simulink model "HTSE_electrolyzer_1MW_DC"  (R2020b)
settings: Solver=ode15s  StartTime=0.0  StopTime=3600*1
model workspace: external: MAT-File (data not in the file)
values from neighbouring files (symbols this model uses):
  Acsflow_aHR = Ltubet * tubenodewidth_aHR    [Electrolyzer_load.m]
  Acsflow_wHR = Ltubet * tubenodewidth_wHR    [Electrolyzer_load.m]
  Anode_aHR = pi*Dtubeo*tubenodewidth_aHR*ntubes    (= 5.35151053616)    [Electrolyzer_load.m]
  Anode_wHR = pi*Dtubeo*tubenodewidth_wHR*ntubes    (= 2.79287586904)    [Electrolyzer_load.m]
  C1 = C1par(4,4)    [tubebankpar.m]
  Cp_I = 500    [Electrolyzer_load.m]
  Cp_S = 500    [Electrolyzer_load.m]
  Dtubei = 0.015748    [Electrolyzer_load.m]
  Dtubeo = Dtubei +2*ttube    (= 0.021336)    [Electrolyzer_load.m]
  dx_cell = L_cell/n_cell    (= 0.0125)    [Electrolyzer_load.m]
  eps_I = 0.1    [Electrolyzer_load.m]
  eps_S = 0.8    [Electrolyzer_load.m]
  F = 96485.33    [Electrolyzer_load.m]    (also in localcur.m = params(6*n+2))
  H2concSS = [9.66170610517 15.4200127744 21.0651099255 26.4111027106 31.267340431 36.180096143 39.6625030093 45.9597835644]    [concSS.mat]
  H2OconcSS = [46.3863122499 40.6280055806 34.9829084296 29.6369156445 24.7806779241 19.8679222121 16.3855153458 10.0882347907]    [concSS.mat]
  h_A = 0.001    [Electrolyzer_load.m]
  h_C = 0.001    [Electrolyzer_load.m]
  h_I = 7.5e-4    (= 0.00075)    [Electrolyzer_load.m]
  h_S = t_C + t_E + t_A    (= 0.00034)    [Electrolyzer_load.m]
  k_A = (Nu_A*lam_A)/dh_A    (= 107.851842105)    [Electrolyzer_load.m]
  k_C = (Nu_C*lam_C)/dh_C    (= 303.235614035)    [Electrolyzer_load.m]
  ktube = 60.5    [Electrolyzer_load.m]
  L_cell = 0.1    [Electrolyzer_load.m]
  lam_I = 25    [Electrolyzer_load.m]
  lam_S = 2    [Electrolyzer_load.m]
  m = mpar(4,4)    [tubebankpar.m]
  MM_H2 = 2    [Electrolyzer_load.m]
  MM_H2O = 18    [Electrolyzer_load.m]
  MM_N2 = 28    [Electrolyzer_load.m]
  MM_O2 = 32    [Electrolyzer_load.m]
  N2concSS = [42.0361226095 42.0361226095 42.0361226095 42.0361226095 42.0361226095 42.0361226095 42.0361226095 42.0361226095]    [concSS.mat]
  n_cell = 8    [Electrolyzer_load.m]
  nhx_aHR = 31    [Electrolyzer_load.m]
  nhx_wHR = 15    [Electrolyzer_load.m]
  ntubes = 500    [Electrolyzer_load.m]
  num_cells = 605711/100    (= 6057.11)    [Electrolyzer_load.m]
  O2concSS = [15.418006168 17.4148227344 19.3723814677 21.2262193353 22.9102241109 24.6138277145 25.8214271218 28.005144464]    [concSS.mat]
  Ppa = 5e5    (= 500000)    [Electrolyzer_load.m]
  rho_I = 8000    [Electrolyzer_load.m]
  rho_S = 5900    [Electrolyzer_load.m]
  sig = 5.6703e-8    (= 5.6703e-08)    [Electrolyzer_load.m]
  St = StD*Dtubeo    (= 0.042672)    [Electrolyzer_load.m]
  T_aSHout = 700 + 273.13    (= 973.13)    [Electrolyzer_load.m]
  T_cell_init = 1073    [Electrolyzer_load.m]
  T_wSHout = 700 + 273.13    (= 973.13)    [Electrolyzer_load.m]
  ttube = 0.002794    [Electrolyzer_load.m]
  V_shell_aHR = (Acsflow_aHR*Ltubel) - (pi*(Dtubeo/2)^2*tubenodewidth_aHR*ntubes)    [Electrolyzer_load.m]
  V_shell_wHR = (Acsflow_wHR*Ltubel) - (pi*(Dtubeo/2)^2*tubenodewidth_wHR*ntubes)    [Electrolyzer_load.m]
  V_tubes_aHR = pi*(Dtubei/2)^2*tubenodewidth_aHR*ntubes    (= 0.0155508525335)    [Electrolyzer_load.m]
  V_tubes_wHR = pi*(Dtubei/2)^2*tubenodewidth_wHR*ntubes    (= 0.00811576479021)    [Electrolyzer_load.m]
  W_cell = 0.0855    [Electrolyzer_load.m]
  x0 = zeros((5*n_cell),1)    [Electrolyzer_load.m]    (also in eqsolver.m = zeros((5*n),1))
libraries: pid_lib x1
settings Model: Creator=jimmonen  LastModifiedBy=jimmonen

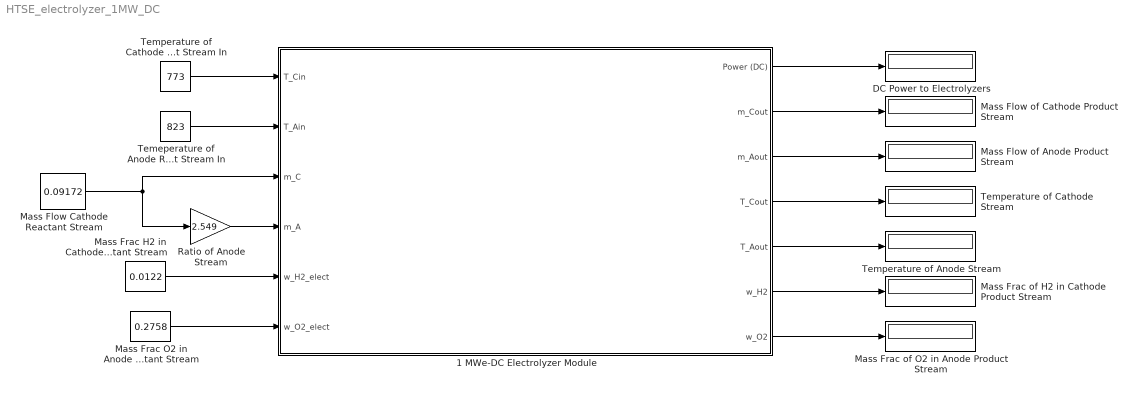
== system HTSE_electrolyzer_1MW_DC ==
  1 MWe-DC Electrolyzer Module : Subsystem
      mask Display: image('G:\My Drive\3. Research\6. HTSE - Detailed Plant\Paper\Figures\SH-FHTSE-1 MW Module.drawio.png'); % Use "Edit Image" on toolstrip to change.
  DC Power to Electrolyzers : Display
  Mass Flow Cathode Reactant Stream : Constant  Value=0.09172
  Mass Flow of Anode Product Stream : Display
  Mass Flow of Cathode Product Stream : Display
  Mass Frac H2 in Cathode Reactant Stream : Constant  Value=0.0122
  Mass Frac O2 in Anode Reactant Stream : Constant  Value=0.2758
  Mass Frac of H2 in Cathode Product Stream : Display
  Mass Frac of O2 in Anode Product Stream : Display
  Ratio of Anode Stream : Gain  Gain=2.549
  Temeperature of Anode Reactant Stream In : Constant  Value=823
  Temperature of Anode Stream : Display
  Temperature of Cathode Reactant Stream In : Constant  Value=773
  Temperature of Cathode Stream : Display
  wires:
  Mass Frac H2 in Cathode Reactant Stream/1 -> 1 MWe-DC Electrolyzer Module/5(w_H2_elect)
  Mass Frac O2 in Anode Reactant Stream/1 -> 1 MWe-DC Electrolyzer Module/6(w_O2_elect)
  Ratio of Anode Stream/1 -> 1 MWe-DC Electrolyzer Module/4(m_A)
  Temperature of Cathode Reactant Stream In/1 -> 1 MWe-DC Electrolyzer Module/1(T_Cin)
  Mass Flow Cathode Reactant Stream/1 -> Ratio of Anode Stream/1, 1 MWe-DC Electrolyzer Module/3(m_C)
  Temeperature of Anode Reactant Stream In/1 -> 1 MWe-DC Electrolyzer Module/2(T_Ain)
  1 MWe-DC Electrolyzer Module/1(Power (DC)) -> DC Power to Electrolyzers/1
  1 MWe-DC Electrolyzer Module/2(m_Cout) -> Mass Flow of Cathode Product Stream/1
  1 MWe-DC Electrolyzer Module/3(m_Aout) -> Mass Flow of Anode Product Stream/1
  1 MWe-DC Electrolyzer Module/6(w_H2) -> Mass Frac of H2 in Cathode Product Stream/1
  1 MWe-DC Electrolyzer Module/7(w_O2) -> Mass Frac of O2 in Anode Product Stream/1
  1 MWe-DC Electrolyzer Module/4(T_Cout) -> Temperature of Cathode Stream/1
  1 MWe-DC Electrolyzer Module/5(T_Aout) -> Temperature of Anode Stream/1

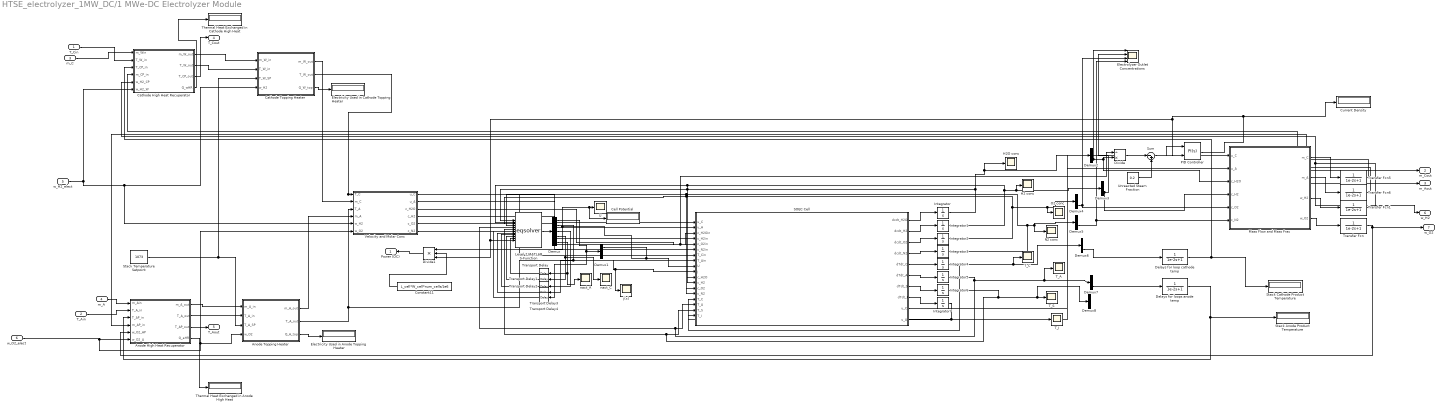
== system HTSE_electrolyzer_1MW_DC/1 MWe-DC Electrolyzer Module ==
  T_Cin : Inport
  T_Ain : Inport  Port=2
  m_C : Inport  Port=3
  m_A : Inport  Port=4
  w_H2_elect : Inport  Port=5
  w_O2_elect : Inport  Port=6
  " SOEC Cell" : MATLAB Function  TreatAsAtomicUnit=on
  Anode High Heat Recuperator : Subsystem
  Anode Topping Heater : MATLAB Function  TreatAsAtomicUnit=on
  Cathode High Heat Recuperator : Subsystem
  Cathode Topping Heater : MATLAB Function  TreatAsAtomicUnit=on
  Cell Potential : Display
  Constant11 : Constant  Value=L_cell*W_cell*num_cells/1e6
  Current Density : Display
  Delays for loop cathode temp : TransferFcn  Denominator=[1e-2 1]
  Delays for loops anode temp : TransferFcn  Denominator=[1e-2 1]
  Demux : Demux  Outputs=[n_cell n_cell n_cell n_cell n_cell ]
  Demux1 : Demux  Outputs=[1 n_cell-1]
  Demux{2..8} (7 alike) : Demux  Outputs=[n_cell-1 1]
  Divide : Product  Inputs=/*
  Divide1 : Product  Inputs=***
  Electricity Used in Anode Topping Heater : Display
  Electricity Used in Cathode Topping Heater : Display
  Electrolyzer Outlet Concentrations : Scope  NumInputPorts=4
  H2 conc : Scope
  H2O conc : Scope
  Integrator : Integrator  InitialCondition=H2OconcSS
  Integrator1 : Integrator  InitialCondition=H2concSS
  Integrator2 : Integrator  InitialCondition=O2concSS
  Integrator3 : Integrator  InitialCondition=N2concSS
  Integrator{4..7} (4 alike) : Integrator  InitialCondition=T_cell_init*ones(n_cell,1)
  Level-2 MATLAB S-Function : M-S-Function  FunctionName=eqsolver  Parameters=n_cell, F, R, t_C, t_E, t_A, sig_C, sig_A, sig_E, A_C, A_A, E_C, E_A, Deff_C, Deff_A, alph, Ppa
  Mass Flow and Mass Frac : MATLAB Function  TreatAsAtomicUnit=on
  N2 conc : Scope
  O2 conc : Scope
  PID Controller : pid_lib/PID Controller  Controller=PI  Form=Parallel  TimeDomain=Continuous-time  UseExternalTs=off  SampleTime=-1  IntegratorMethod=Forward Euler  FilterMethod=Forward Euler  ControllerParametersSource=internal  P=30  I=-12.5  D=0  UseFilter=on  N=100  TunerSelectOption=Transfer Function Based (PID Tuner App)  InitialConditionSource=internal  InitialConditionForIntegrator=15000  InitialConditionForFilter=0  DifferentiatorICPrevScaledInput=0  ExternalReset=none  TrackingMode=on  Kt=1  LimitOutput=on  SatLimitsSource=internal  UpperSaturationLimit=15000  LowerSaturationLimit=0  LinearizeAsGain=on  AntiWindupMode=none  Kb=1  POutMin=[]  POutMax=[]  IOutMin=[]  IOutMax=[]  DOutMin=[]  DOutMax=[]  NOutMin=[]  NOutMax=[]  SumOutMin=[]  SumOutMax=[]  SaturationOutMin=[]  SaturationOutMax=[]  PParamMin=[]  PParamMax=[]  IParamMin=[]  IParamMax=[]  DParamMin=[]  DParamMax=[]  NParamMin=[]  NParamMax=[]  KbParamMin=[]  KbParamMax=[]  KtParamMin=[]  KtParamMax=[]  KbOutMin=[]  KbOutMax=[]  KtOutMin=[]  KtOutMax=[]  IntegratorOutMin=[]  IntegratorOutMax=[]  FilterOutMin=[]  FilterOutMax=[]  SumI1OutMin=[]  SumI1OutMax=[]  SumI2OutMin=[]  SumI2OutMax=[]  SumI3OutMin=[]  SumI3OutMax=[]  SumI4OutMin=[]  SumI4OutMax=[]  SumDOutMin=[]  SumDOutMax=[]  DifferentiatorOutMin=[]  DifferentiatorOutMax=[]  FilterDiffOutCoefMin=[]  FilterDiffOutCoefMax=[]  ReciprocalOutMin=[]  ReciprocalOutMax=[]  SumDenOutMin=[]  SumDenOutMax=[]  SumNumOutMin=[]  SumNumOutMax=[]  DivideOutMin=[]  DivideOutMax=[]  UdiffTsProdOutMin=[]  UdiffTsProdOutMax=[]  NTsProdOutMin=[]  NTsProdOutMax=[]  UintegralTsProdOutMin=[]  UintegralTsProdOutMax=[]  UngainTsProdOutMin=[]  UngainTsProdOutMax=[]  IntegratorContinuousStateAttributes=''  IntegratorStateMustResolveToSignalObject=off  IntegratorRTWStateStorageClass=Auto  FilterContinuousStateAttributes=''  FilterStateMustResolveToSignalObject=off  FilterRTWStateStorageClass=Auto  ParallelPVariant=InternalParameters  IdealPVariant=Disabled  IVariant=InternalParameters  DVariant=Disabled  IntegratorVariant=Continuous  SatVariant=Enabled  AWVariant=Passthrough  PCopyVariant=Disabled  TRVariant=Enabled  FdbkBlocksVariant=Forward  IdealPFdbkVariant=Disabled  SatFdbkVariant=Disabled  DerivativeFilterVariant=Disabled  NVariant=Disabled  NCopyVariant=Disabled_SignalSpec  FilterICVariant=Disabled  IntegratorICVariant=InternalICs  ExternalResetVariant=Disabled  TRSumVariant=TrackingMode  SumFdbkVariant=Disabled  SumVariant=Sum_PI  TsampFilterVariant=InternalTs  TsampNgainVariant=Passthrough  TsampIntegralVariant=Passthrough  ExternalSaturationOutDataTypeStr=Inherit: Same as second input
  Stack Anode Product Temperature : Display
  Stack Cathode Product Temperature : Display
  Stack Temperature Setpoint : Constant  Value=1073
  Sum : Sum  Inputs=|-+
  T_A : Scope
  T_C : Scope
  T_I : Scope
  T_S : Scope
  Thermal Heat Exchanged in Anode High Heat : Display
  Thermal Heat Exchanged in Cathode High Heat : Display
  Transfer Fcn{,1,5..6} (4 alike) : TransferFcn  Denominator=[1e-2 1]
  Transport Delay : TransportDelay  DelayTime=0.1  InitialOutput=x0(4*n_cell+1:end)
  Transport Delay1 : TransportDelay  DelayTime=0.1  InitialOutput=x0(3*n_cell+1:4*n_cell)
  Transport Delay2 : TransportDelay  DelayTime=0.1  InitialOutput=x0(2*n_cell+1:3*n_cell)
  Transport Delay3 : TransportDelay  DelayTime=0.1  InitialOutput=x0(n_cell+1:2*n_cell)
  Transport Delay4 : TransportDelay  DelayTime=0.1  InitialOutput=x0(1:n_cell)
  U : Scope
  Unreacted Steam Fraction : Constant  Value=0.2
  Velocity and Molar Conc : MATLAB Function  TreatAsAtomicUnit=on
  j(x) : Scope
  nact_A : Scope
  nact_C : Scope
  Power (DC) : Outport
  m_Cout : Outport  Port=2
  m_Aout : Outport  Port=3
  T_Cout : Outport  Port=4
  T_Aout : Outport  Port=5
  w_H2 : Outport  Port=6
  w_O2 : Outport  Port=7
  wires:
  " SOEC Cell"/2(dcdt_H2) -> Integrator1/1
  " SOEC Cell"/7(dTdt_S) -> Integrator6/1
  " SOEC Cell"/3(dcdt_O2) -> Integrator2/1
  Divide1/1 -> Power (DC)/1
  " SOEC Cell"/5(dTdt_C) -> Integrator4/1
  Demux6/2 -> Delays for loop cathode temp/1
  Integrator4/1 -> Demux6/1, T_C/1, " SOEC Cell"/15(T_C)
  Integrator7/1 -> " SOEC Cell"/18(T_I), T_I/1
  " SOEC Cell"/8(dTdt_I) -> Integrator7/1
  Demux2/2 -> Divide/2, Mass Flow and Mass Frac/3(c_H2O), Electrolyzer Outlet Concentrations/1
  " SOEC Cell"/4(dcdt_N2) -> Integrator3/1
  " SOEC Cell"/6(dTdt_A) -> Integrator5/1
  Divide/1 -> Sum/1
  Sum/1 -> PID Controller/1
  Constant11/1 -> Divide1/2
  Demux7/2 -> Delays for loops anode temp/1
  " SOEC Cell"/1(dcdt_H2O) -> Integrator/1
  Demux4/2 -> Electrolyzer Outlet Concentrations/3, Mass Flow and Mass Frac/5(c_O2)
  Demux5/2 -> Electrolyzer Outlet Concentrations/4, Mass Flow and Mass Frac/6(c_N2)
  Mass Flow and Mass Frac/1(m_C) -> Transfer Fcn5/1
  Mass Flow and Mass Frac/2(m_A) -> Transfer Fcn6/1
  " SOEC Cell"/9(u_C) -> Mass Flow and Mass Frac/1(u_C)
  " SOEC Cell"/10(u_A) -> Mass Flow and Mass Frac/2(u_A)
  Mass Flow and Mass Frac/4(w_O2) -> Transfer Fcn/1
  Mass Flow and Mass Frac/3(w_H2) -> Transfer Fcn1/1
  w_H2_elect/1 -> Cathode Topping Heater/4(w_H2), Velocity and Molar Conc/5(w_H2), Cathode High Heat Recuperator/6(w_H2_W)
  w_O2_elect/1 -> Velocity and Molar Conc/6(w_O2), Anode Topping Heater/4(w_O2), Anode High Heat Recuperator/6(w_O2_A)
  Velocity and Molar Conc/1(u_C) -> " SOEC Cell"/1("u_C ")
  Velocity and Molar Conc/2(u_A) -> " SOEC Cell"/2("u_A ")
  Velocity and Molar Conc/3(c_H2O) -> Divide/1, " SOEC Cell"/3(c_H2Oin)
  Velocity and Molar Conc/4(c_H2) -> " SOEC Cell"/4(c_H2in)
  Velocity and Molar Conc/5(c_O2) -> " SOEC Cell"/5(c_O2in)
  Velocity and Molar Conc/6(c_N2) -> " SOEC Cell"/6(c_N2in)
  Transfer Fcn/1 -> Anode High Heat Recuperator/5(w_O2_AP), w_O2/1
  Transfer Fcn1/1 -> w_H2/1, Cathode High Heat Recuperator/5(w_H2_CP)
  Demux/2 -> Transport Delay3/1, " SOEC Cell"/10(j), j(x)/1
  Integrator1/1 -> Level-2 MATLAB S-Function/2, " SOEC Cell"/12(c_H2), Demux3/1, H2 conc/1
  Integrator/1 -> Demux2/1, H2O conc/1, Level-2 MATLAB S-Function/1, " SOEC Cell"/11(c_H2O)
  Transport Delay3/1 -> Level-2 MATLAB S-Function/8
  Demux/3 -> Transport Delay2/1
  Demux/1 -> Transport Delay4/1, Demux1/1
  Integrator5/1 -> Level-2 MATLAB S-Function/5, " SOEC Cell"/16(T_A), Demux7/1, T_A/1
  Level-2 MATLAB S-Function/1 -> Demux/1
  Demux/5 -> Transport Delay/1, nact_A/1
  Demux/4 -> Transport Delay1/1, nact_C/1
  Transport Delay2/1 -> Level-2 MATLAB S-Function/9
  Transport Delay4/1 -> Level-2 MATLAB S-Function/7
  Transport Delay1/1 -> Level-2 MATLAB S-Function/10
  Transport Delay/1 -> Level-2 MATLAB S-Function/11
  Integrator2/1 -> Level-2 MATLAB S-Function/3, " SOEC Cell"/13(c_O2), Demux4/1, O2 conc/1
  Demux1/1 -> Cell Potential/1, U/1, Divide1/1, " SOEC Cell"/9(U)
  Demux3/2 -> Electrolyzer Outlet Concentrations/2, Mass Flow and Mass Frac/4(c_H2)
  Cathode High Heat Recuperator/2(T_W_out) -> Cathode Topping Heater/2(T_W_in)
  Cathode High Heat Recuperator/1(m_W_out) -> Cathode Topping Heater/1(m_W_in)
  Stack Temperature Setpoint/1 -> Anode Topping Heater/3(T_A_SP), Cathode Topping Heater/3(T_W_SP)
  m_C/1 -> Cathode High Heat Recuperator/1("m_Win ")
  T_Cin/1 -> Cathode High Heat Recuperator/2(T_W_in)
  Cathode Topping Heater/1(m_W_out) -> Velocity and Molar Conc/2(m_C)
  m_A/1 -> Anode High Heat Recuperator/1("m_Ain ")
  T_Ain/1 -> Anode High Heat Recuperator/2(T_A_in)
  Anode Topping Heater/1(m_A_out) -> Velocity and Molar Conc/4(m_A)
  Anode Topping Heater/2(T_A_out) -> Velocity and Molar Conc/3(T_A), " SOEC Cell"/8(T_Ain)
  Anode High Heat Recuperator/1(m_A_out) -> Anode Topping Heater/1(m_A_in)
  Delays for loop cathode temp/1 -> Cathode High Heat Recuperator/3(T_CP_in), Stack Cathode Product Temperature/1
  Delays for loops anode temp/1 -> Stack Anode Product Temperature/1, Anode High Heat Recuperator/3(T_AP_in)
  Transfer Fcn5/1 -> m_Cout/1, Cathode High Heat Recuperator/4("m_CP_in ")
  Transfer Fcn6/1 -> m_Aout/1, Anode High Heat Recuperator/4("m_AP_in ")
  PID Controller/1 -> PID Controller/2, Level-2 MATLAB S-Function/12, Divide1/3, Current Density/1
  Unreacted Steam Fraction/1 -> Sum/2
  Integrator6/1 -> Demux8/1, T_S/1, Level-2 MATLAB S-Function/6, " SOEC Cell"/17(T_S)
  Cathode Topping Heater/2(T_W_out) -> " SOEC Cell"/7(T_Cin), Velocity and Molar Conc/1(T_C)
  Integrator3/1 -> Demux5/1, N2 conc/1, Level-2 MATLAB S-Function/4, " SOEC Cell"/14(c_N2)
  Anode High Heat Recuperator/2(T_A_out) -> Anode Topping Heater/2(T_A_in)
  Cathode High Heat Recuperator/3(T_CP_out) -> T_Cout/1
  Cathode High Heat Recuperator/4(Q_wHR) -> Thermal Heat Exchanged in Cathode High Heat/1
  Cathode Topping Heater/3(Q_W_top) -> Electricity Used in Cathode Topping Heater/1
  Anode Topping Heater/3(Q_A_top) -> Electricity Used in Anode Topping Heater/1
  Anode High Heat Recuperator/3(T_AP_out) -> T_Aout/1
  Anode High Heat Recuperator/4(Q_aHR) -> Thermal Heat Exchanged in Anode High Heat/1

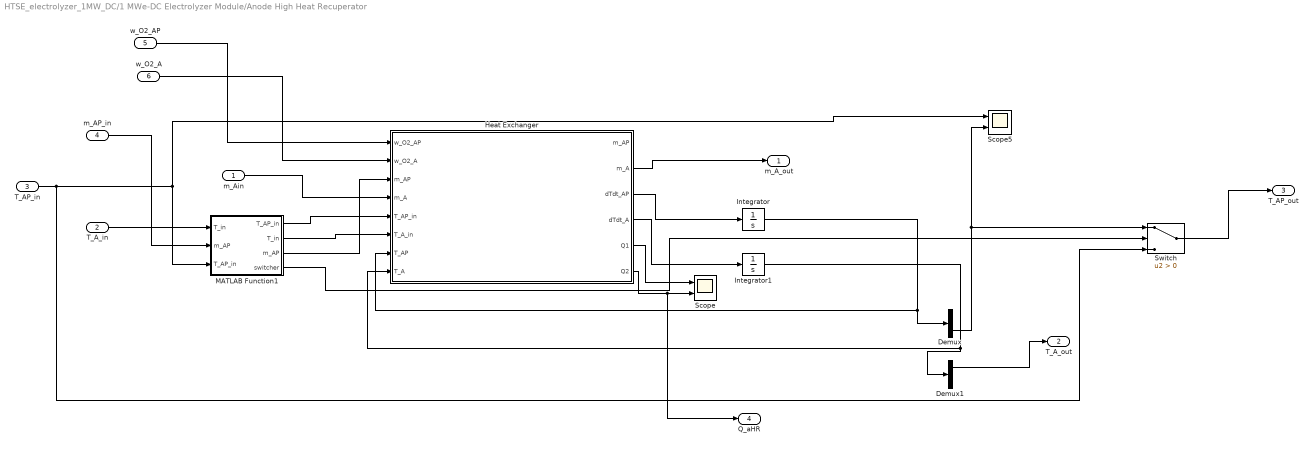
== system HTSE_electrolyzer_1MW_DC/1 MWe-DC Electrolyzer Module/Anode High Heat Recuperator ==
  "m_Ain " : Inport
  T_A_in : Inport  Port=2
  T_AP_in : Inport  Port=3
  "m_AP_in " : Inport  Port=4
  w_O2_AP : Inport  Port=5
  w_O2_A : Inport  Port=6
  Demux : Demux  Outputs=[nhx_aHR-1 1]
  Demux1 : Demux  Outputs=[1 nhx_aHR-1]
  Heat Exchanger : MATLAB Function  TreatAsAtomicUnit=on
  Integrator : Integrator  InitialCondition=ones(nhx_aHR, 1)*(T_aSHout)
  Integrator1 : Integrator  InitialCondition=ones(nhx_aHR, 1)*(T_aSHout)
  MATLAB Function1 : MATLAB Function  TreatAsAtomicUnit=on
  Scope : Scope  NumInputPorts=2
  Scope5 : Scope  NumInputPorts=2
  Switch : Switch  Criteria=u2 > Threshold
  m_A_out : Outport
  T_A_out : Outport  Port=2
  T_AP_out : Outport  Port=3
  Q_aHR : Outport  Port=4
  wires:
  Integrator1/1 -> Demux1/1, Heat Exchanger/8(T_A)
  "m_AP_in "/1 -> MATLAB Function1/2("m_AP ")
  Demux/2 -> Scope5/2, Switch/1
  Integrator/1 -> Demux/1, Heat Exchanger/7(T_AP)
  "m_Ain "/1 -> Heat Exchanger/4("m_A ")
  Heat Exchanger/4(dTdt_A) -> Integrator1/1
  Heat Exchanger/3(dTdt_AP) -> Integrator/1
  T_AP_in/1 -> Switch/3, Scope5/1, MATLAB Function1/3("T_AP_in ")
  Heat Exchanger/5(Q1) -> Scope/1
  MATLAB Function1/3(m_AP) -> Heat Exchanger/3("m_AP ")
  MATLAB Function1/2(T_in) -> Heat Exchanger/6(T_A_in)
  MATLAB Function1/1(T_AP_in) -> Heat Exchanger/5(T_AP_in)
  Demux1/1 -> T_A_out/1
  T_A_in/1 -> MATLAB Function1/1("T_in ")
  MATLAB Function1/4(switcher) -> Switch/2
  Switch/1 -> T_AP_out/1
  Heat Exchanger/6(Q2) -> Q_aHR/1, Scope/2
  Heat Exchanger/2(m_A) -> m_A_out/1
  w_O2_AP/1 -> Heat Exchanger/1(w_O2_AP)
  w_O2_A/1 -> Heat Exchanger/2(w_O2_A)

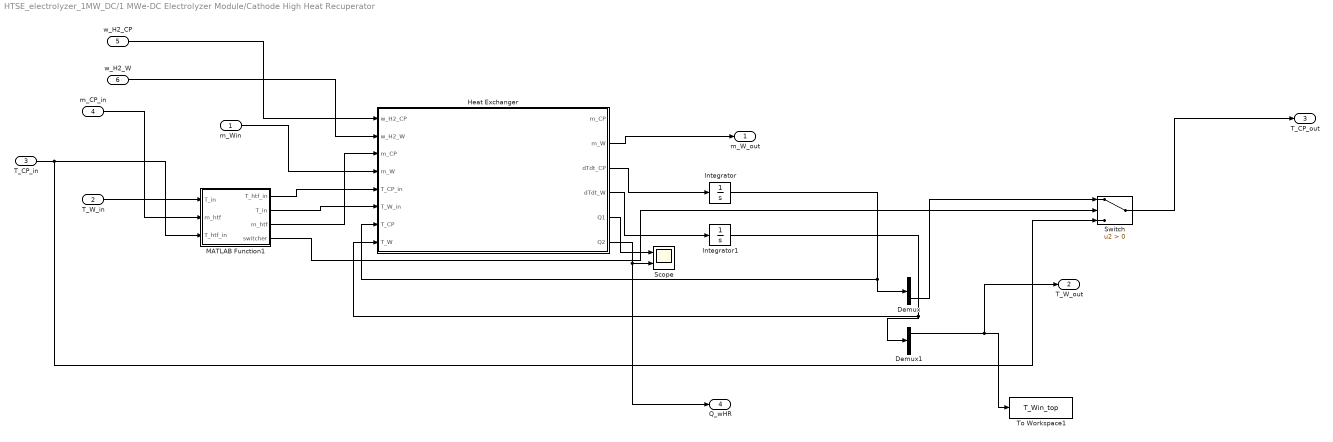
== system HTSE_electrolyzer_1MW_DC/1 MWe-DC Electrolyzer Module/Cathode High Heat Recuperator ==
  "m_Win " : Inport
  T_W_in : Inport  Port=2
  T_CP_in : Inport  Port=3
  "m_CP_in " : Inport  Port=4
  w_H2_CP : Inport  Port=5
  w_H2_W : Inport  Port=6
  Demux : Demux  Outputs=[nhx_wHR-1 1]
  Demux1 : Demux  Outputs=[1 nhx_wHR-1]
  Heat Exchanger : MATLAB Function  TreatAsAtomicUnit=on
  Integrator : Integrator  InitialCondition=ones(nhx_wHR, 1)*(T_wSHout)
  Integrator1 : Integrator  InitialCondition=ones(nhx_wHR, 1)*(T_wSHout)
  MATLAB Function1 : MATLAB Function  TreatAsAtomicUnit=on
  Scope : Scope  NumInputPorts=2
  Switch : Switch  Criteria=u2 > Threshold
  To Workspace1 : ToWorkspace  VariableName=T_Win_top  SaveFormat=Timeseries  SampleTime=-1
  m_W_out : Outport
  T_W_out : Outport  Port=2
  T_CP_out : Outport  Port=3
  Q_wHR : Outport  Port=4
  wires:
  Integrator1/1 -> Demux1/1, Heat Exchanger/8(T_W)
  "m_CP_in "/1 -> MATLAB Function1/2("m_htf ")
  Demux/2 -> Switch/1
  Integrator/1 -> Demux/1, Heat Exchanger/7(T_CP)
  "m_Win "/1 -> Heat Exchanger/4("m_W ")
  Heat Exchanger/4(dTdt_W) -> Integrator1/1
  Heat Exchanger/3(dTdt_CP) -> Integrator/1
  T_CP_in/1 -> Switch/3, MATLAB Function1/3("T_htf_in ")
  Heat Exchanger/5(Q1) -> Scope/1
  MATLAB Function1/3(m_htf) -> Heat Exchanger/3("m_CP ")
  MATLAB Function1/2(T_in) -> Heat Exchanger/6(T_W_in)
  MATLAB Function1/1(T_htf_in) -> Heat Exchanger/5(T_CP_in)
  Demux1/1 -> T_W_out/1, To Workspace1/1
  T_W_in/1 -> MATLAB Function1/1("T_in ")
  MATLAB Function1/4(switcher) -> Switch/2
  Switch/1 -> T_CP_out/1
  Heat Exchanger/6(Q2) -> Q_wHR/1, Scope/2
  Heat Exchanger/2(m_W) -> m_W_out/1
  w_H2_CP/1 -> Heat Exchanger/1(w_H2_CP)
  w_H2_W/1 -> Heat Exchanger/2(w_H2_W)

== matlab function HTSE_electrolyzer_1MW_DC/1 MWe-DC Electrolyzer Module/Mass Flow and Mass Frac ==
  data: u_C input; u_A input; c_H2O input; c_H2 input; c_O2 input; c_N2 input; num_cells parameter; MM_H2O parameter; h_A parameter; W_cell parameter; h_C parameter; MM_O2 parameter; m_C output; m_A output; w_H2 output; MM_N2 parameter; MM_H2 parameter; w_O2 output
function [m_C, m_A, w_H2, w_O2] = conc_to_mass(u_C, u_A, c_H2O, c_H2, c_O2, c_N2, num_cells, MM_H2O,h_A, W_cell, h_C, MM_O2, MM_N2, MM_H2)

%mass flows cathode
m_H2O = u_C*h_C*W_cell*MM_H2O*c_H2O*num_cells/1000;
m_H2 =  u_C*h_C*W_cell*MM_H2*c_H2*num_cells/1000;
m_C = m_H2O + m_H2;


%mass fractions cathode
w_H2O = m_H2O/(m_H2O + m_H2);
w_H2 = 1 - w_H2O;

%mass flows anode
m_O2 = u_A*h_A*W_cell*MM_O2*c_O2*num_cells/1000;
m_N2 = u_A*h_A*W_cell*MM_N2*c_N2*num_cells/1000;
m_A = (m_O2 + m_N2);

%mass fractions anode
w_O2 = m_O2/(m_O2 + m_N2);

== matlab function HTSE_electrolyzer_1MW_DC/1 MWe-DC Electrolyzer Module/Cathode High Heat Recuperator/Heat Exchanger ==
  data: w_H2_CP input; w_H2_W input; m_CP input; m_W input; T_CP_in input; T_W_in input; T_CP input; m_CP output; m_W output; T_W input; dTdt_CP output; dTdt_W output; V_shell_wHR parameter; V_tubes_wHR parameter; nhx_wHR parameter; Acsflow_wHR parameter; St parameter; Dtubei parameter; ntubes parameter; C1 parameter; m parameter; ktube parameter; ttube parameter; Dtubeo parameter; Anode_wHR parameter; Q1 output; Q2 output
function [m_CP, m_W, dTdt_CP, dTdt_W, Q1, Q2]   = HX(w_H2_CP, w_H2_W, m_CP, m_W, T_CP_in,  ...
    T_W_in, T_CP, T_W, V_shell_wHR, V_tubes_wHR, nhx_wHR,...
    Acsflow_wHR, St, Dtubei, ntubes, C1, m, ktube, ttube, Dtubeo, Anode_wHR)

%% Properties

T_CP_avg = (T_CP_in + T_CP(end))/2;
w_H2O_CP = 1 - w_H2_CP;

[rho_H2O1, mu_H2O1, k_H2O1, C_H2O1] = water(T_CP_avg);
[rho_H21, mu_H21, k_H21, C_H21] = hydrogen(T_CP_avg);

%use weight fractions for mixing of properties
[rho_CP, mu_CP, k_CP, C_CP] = prop_mix(rho_H2O1, rho_H21, mu_H2O1, mu_H21, k_H2O1, k_H21, C_H2O1, C_H21, w_H2O_CP, w_H2_CP);

% Steam Properties
T_W_avg = (T_W_in + T_W(1))/2;
w_H2O_W = 1 - w_H2_W;

[rho_H2O2, mu_H2O2, k_H2O2, C_H2O2] = water(T_W_avg);
[rho_H22, mu_H22, k_H22, C_H22] = hydrogen(T_W_avg);

%use weight fractions for mixing of properties
[rho_W, mu_W, k_W, C_W] = prop_mix(rho_H2O2, rho_H22, mu_H2O2, mu_H22, k_H2O2, k_H22, C_H2O2, C_H22, w_H2O_W, w_H2_W);


%% Heat Transfer Coefficient Calcs

%CP is in shell

Pr_CP = C_CP*mu_CP/k_CP; %Prandtl # for CP, flow in pipe

%Determining the Reynolds # of the HTF using the maximum velocity through
%bank of tubes
v_CP = m_CP/(Acsflow_wHR*rho_CP); %m/s, velocity before hitting any tubes
vmax_CP = (St*v_CP)/(St-Dtubeo);
Remax_CP = (rho_CP*vmax_CP*Dtubeo)/mu_CP; %max reynolds number based on diameter and flow in between tubes
Nu_CP = 1.13*C1 * Remax_CP^m * Pr_CP^(1/3);

h_CP = Nu_CP*k_CP/Dtubeo; %convection ht coefficient for htf in crossflow over a bank of tubes
                            %W/m^2*K

%==========================================================================
% Steam is in tubes

m_W = m_W/ntubes; %kg/s, divide flow up into each tube for Re calcs

v_W = m_W/(rho_W*pi*(Dtubei/2)^2);
Re_W = (rho_W*v_W*Dtubei)/mu_W; %Reynolds # for HTF, flow in pipe
Pr_W = C_W*mu_W/k_W; %Prandtl # for HTF, flow in pipe

%HT coef for turbulent flow in ciruclar tube, i.e. high Re#
h_W = 0.023*Re_W^0.8*Pr_W^0.4*k_W/(Dtubei); %W/(m^2*K)

%HT coef for laminar flow
if Re_W < 2000
    h_W = 4.36*k_W/(Dtubei); %W/(m^2*K)
end

%to be used in energy bal/ODE on HTF
%from Incroprera et al., pg 507&514


%calculating overall heat transfer coefficient using thermal resistance,
%ignores effects of fins and fouling

U = ( (1/h_CP) + (1/h_W) + (ttube/ktube) )^-1; %overall ht coef, W/m^2*K 

%% Energy Balance

%initializing each energybal as zero to define size of each column vector

dTdt_CP = zeros(size(T_CP));
dTdt_W = zeros(size(T_W));

%HTF energy balance
dTdt_CP(1) = (m_CP*C_CP*(T_CP_in - T_CP(1)) - U*Anode_wHR * (T_CP(1) - T_W(1)))/(V_shell_wHR*rho_CP*C_CP);
dTdt_CP(2:nhx_wHR) = (m_CP*C_CP*(T_CP(1:nhx_wHR-1) - T_CP(2:nhx_wHR)) - U*Anode_wHR * (T_CP(2:nhx_wHR) - T_W(2:nhx_wHR)))/(V_shell_wHR*rho_CP*C_CP);

m_W = m_W*ntubes; %Recombining flow for energy balance

%Energy balance, counter flow
dTdt_W(nhx_wHR) = (m_W*C_W*(T_W_in - T_W(nhx_wHR)) + U*Anode_wHR *(T_CP(nhx_wHR) - T_W(nhx_wHR)))/(V_tubes_wHR*rho_W*C_W);
dTdt_W(1:nhx_wHR-1) = (m_W*C_W*(T_W(2:nhx_wHR) - T_W(1:nhx_wHR-1)) + U*Anode_wHR * (T_CP(1:nhx_wHR-1) - T_W(1:nhx_wHR-1)))/(V_tubes_wHR*rho_W*C_W);


Q1 = (m_CP*C_CP*(T_CP_in - T_CP(nhx_wHR)))/1e6;
Q2 = -(m_W*C_W*(T_W_in - T_W(1)))/1e6;

if Q1 < 0
    Q1 = 0;
end



end

== matlab function HTSE_electrolyzer_1MW_DC/1 MWe-DC Electrolyzer Module/Cathode High Heat Recuperator/MATLAB Function1 ==
  data: T_htf_in output; T_in input; T_in output; m_htf input; T_htf_in input; m_htf output; switcher output
function [T_htf_in, T_in, m_htf, switcher] = HXbypass(T_in, m_htf, T_htf_in)

if T_htf_in < T_in
    m_htf = 0;
    switcher = 0;
else 
    switcher = 1;
end

== matlab function HTSE_electrolyzer_1MW_DC/1 MWe-DC Electrolyzer Module/Anode High Heat Recuperator/Heat Exchanger ==
  data: w_O2_AP input; w_O2_A input; m_AP input; m_A input; T_AP_in input; T_A_in input; T_AP input; m_AP output; m_A output; T_A input; dTdt_AP output; dTdt_A output; V_shell_aHR parameter; V_tubes_aHR parameter; nhx_aHR parameter; Acsflow_aHR parameter; St parameter; Dtubei parameter; ntubes parameter; C1 parameter; m parameter; ktube parameter; ttube parameter; Dtubeo parameter; Anode_aHR parameter; Q1 output; Q2 output
function [m_AP, m_A, dTdt_AP, dTdt_A, Q1, Q2]   = HX(w_O2_AP, w_O2_A, m_AP, m_A, T_AP_in,  ...
    T_A_in, T_AP, T_A, V_shell_aHR, V_tubes_aHR, nhx_aHR,...
    Acsflow_aHR, St, Dtubei, ntubes, C1, m, ktube, ttube, Dtubeo, Anode_aHR)

%% Properties

%Anode Product Properties
T_AP_avg = (T_AP_in + T_AP(end))/2;

[rho_oxy1, mu_oxy1, k_oxy1, C_oxy1] = oxygen(T_AP_avg);
[rho_nit1, mu_nit1, k_nit1, C_nit1] = nitrogen(T_AP_avg);

%use weight fractions for mixing of properties
w_N2_AP =  1 - w_O2_AP;
[rho_AP, mu_AP, k_AP, C_AP] = prop_mix(rho_oxy1, rho_nit1, mu_oxy1, mu_nit1, k_oxy1, k_nit1, C_oxy1, C_nit1, w_O2_AP, w_N2_AP);

%Sweep Gas Properties
T_A_avg = (T_A_in + T_A(1))/2;

[rho_oxy2, mu_oxy2, k_oxy2, C_oxy2] = oxygen(T_A_avg);
[rho_nit2, mu_nit2, k_nit2, C_nit2] = nitrogen(T_A_avg);

%use weight fractions for mixing of properties
w_N2_A =  1 - w_O2_A;
[rho_A, mu_A, k_A, C_A] = prop_mix(rho_oxy2, rho_nit2, mu_oxy2, mu_nit2, k_oxy2, k_nit2, C_oxy2, C_nit2, w_O2_A, w_N2_A);

%% Heat Transfer Coefficient Calcs

Pr_AP = C_AP*mu_AP/k_AP; %Prandtl # for AP

%Determining the Reynolds # of the HTF using the maximum velocity through
%bank of tubes
v_AP = m_AP/(Acsflow_aHR*rho_AP); %m/s, velocity before hitting any tubes
vmax_AP = (St*v_AP)/(St-Dtubeo);
Remax_AP = (rho_AP*vmax_AP*Dtubeo)/mu_AP; %max reynolds number based on diameter and flow in between tubes
Nu_AP = 1.13*C1 * Remax_AP^m * Pr_AP^(1/3);

h_AP = Nu_AP*k_AP/Dtubeo; %convection ht coefficient for htf in crossflow over a bank of tubes
                            %W/m^2*K

%==========================================================================
%Air is in tubes
m_A = m_A/ntubes; %kg/s, divide flow up into each tube for Re calcs

v_A = m_A/(rho_A*pi*(Dtubei/2)^2);
Re_A = (rho_A*v_A*Dtubei)/mu_A; %Reynolds # for HTF, flow in pipe
Pr_A = C_A*mu_A/k_A; %Prandtl # for HTF, flow in pipe

%HT coef for crude for turbulent flow in ciruclar tube, i.e. high Re#
h_A = 0.023*Re_A^0.8*Pr_A^0.4*k_A/(Dtubei); %W/(m^2*K)

%HT coef for crude for laminar flow in circular tube, i.e. low Re#
if Re_A < 2000
    h_A = 4.36*k_A/(Dtubei); %W/(m^2*K)
end

%to be used in energy bal/ODE on HTF
%from Incroprera et al., pg 507&514

%calculating overall heat transfer coefficient using thermal resistance,
%ignores effects of fins and fouling

U = ( (1/h_AP) + (1/h_A) + (ttube/ktube) )^-1; %overall ht coef, W/m^2*K 

%% Energy Balance

%initializing each energybal as zero to define size of each column vector

dTdt_AP = zeros(size(T_AP));
dTdt_A = zeros(size(T_A));

%HTF energy balance
dTdt_AP(1) = (m_AP*C_AP*(T_AP_in - T_AP(1)) - U*Anode_aHR * (T_AP(1) - T_A(1)))/(V_shell_aHR*rho_AP*C_AP);
dTdt_AP(2:nhx_aHR) = (m_AP*C_AP*(T_AP(1:nhx_aHR-1) - T_AP(2:nhx_aHR)) - U*Anode_aHR * (T_AP(2:nhx_aHR) - T_A(2:nhx_aHR)))/(V_shell_aHR*rho_AP*C_AP);

m_A = m_A*ntubes; %Recombining flow for energy balance
%Energy balance, counter flow
dTdt_A(nhx_aHR) = (m_A*C_A*(T_A_in - T_A(nhx_aHR)) + U*Anode_aHR *(T_AP(nhx_aHR) - T_A(nhx_aHR)))/(V_tubes_aHR*rho_A*C_A);
dTdt_A(1:nhx_aHR-1) = (m_A*C_A*(T_A(2:nhx_aHR) - T_A(1:nhx_aHR-1)) + U*Anode_aHR * (T_AP(1:nhx_aHR-1) - T_A(1:nhx_aHR-1)))/(V_tubes_aHR*rho_A*C_A);


Q1 = (m_AP*C_AP*(T_AP_in - T_AP(nhx_aHR)))/1e6;
Q2 = -(m_A*C_A*(T_A_in - T_A(1)))/1e6;


if Q1 < 0
    Q1 = 0;
end



end

== matlab function HTSE_electrolyzer_1MW_DC/1 MWe-DC Electrolyzer Module/Anode High Heat Recuperator/MATLAB Function1 ==
  data: T_AP_in output; T_in input; T_in output; m_AP input; T_AP_in input; m_AP output; switcher output
function [T_AP_in, T_in, m_AP, switcher] = HXbypass(T_in, m_AP, T_AP_in)

if T_AP_in < T_in
    m_AP = 0;
    switcher = 0;
else 
    switcher = 1;
end

== matlab function HTSE_electrolyzer_1MW_DC/1 MWe-DC Electrolyzer Module/Anode Topping Heater ==
  data: m_A_in input; m_A_out output; T_A_in input; T_A_out output; T_A_SP input; w_O2 input; Q_A_top output; eta_elec parameter
function [m_A_out, T_A_out, Q_A_top] = toppingheater(m_A_in, T_A_in, T_A_SP, w_O2, eta_elec)

[~, ~, ~, C_O2] = oxygen((T_A_in + T_A_SP)/2);

[~, ~, ~, C_N2] = nitrogen((T_A_in + T_A_SP)/2);

w_N2 = 1 - w_O2;

C_A = C_O2*w_N2 + C_N2*w_O2;

Q_A_top = (m_A_in*C_A*(T_A_SP - T_A_in))/1e6/eta_elec;

if Q_A_top >= 6/1000
    Q_A_top = 6/1000;
    m_A_out = m_A_in;
    T_A_out = (Q_A_top*1e6*eta_elec)/(m_A_in*C_A) + T_A_in;
else
    
    m_A_out = m_A_in;
    T_A_out = T_A_SP;
end

== matlab function HTSE_electrolyzer_1MW_DC/1 MWe-DC Electrolyzer Module/Cathode Topping Heater ==
  data: m_W_in input; m_W_out output; T_W_in input; T_W_out output; T_W_SP input; w_H2 input; Q_W_top output; eta_elec parameter
function [m_W_out, T_W_out, Q_W_top] = toppingheater(m_W_in, T_W_in, T_W_SP, w_H2, eta_elec)

[~, ~, ~, C_H2O] = water((T_W_in + T_W_SP)/2);
[~, ~, ~, C_H2] = hydrogen((T_W_in + T_W_SP)/2);

w_H2O = 1 - w_H2;

C_W = C_H2O*w_H2O + C_H2*w_H2;
Q_W_top = (m_W_in*C_W*(T_W_SP - T_W_in))/1e6/eta_elec;

if Q_W_top >= 25/1000
    Q_W_top = 25/1000;
    m_W_out = m_W_in;
    T_W_out = (Q_W_top*1e6*eta_elec)/(m_W_in*C_W) + T_W_in;
else
    
    m_W_out = m_W_in;
    T_W_out = T_W_SP;
end

== matlab function HTSE_electrolyzer_1MW_DC/1 MWe-DC Electrolyzer Module/Velocity and Molar Conc ==
  data: u_C output; u_A output; T_C input; m_C input; T_A input; m_A input; w_H2 input; w_O2 input; MM_H2O parameter; MM_O2 parameter; MM_H2 parameter; MM_N2 parameter; W_cell parameter; h_C parameter; h_A parameter; num_cells parameter; c_H2O output; c_H2 output; c_O2 output; c_N2 output; Ppa parameter
function [ u_C, u_A, c_H2O, c_H2, c_O2, c_N2] = conc_and_vel(T_C, m_C, T_A, m_A, w_H2, w_O2,...
    MM_H2O, MM_O2, MM_H2, MM_N2, W_cell, h_C, h_A, num_cells, Ppa)


%Ideal Gas Law: n/V = P/RT
R = 8.314; %J/mol-K
c_Tc = Ppa/(R*T_C); %mol/m^3, total concentration cathode stream
c_Ta = Ppa/(R*T_A); %mol/m^3, total concentration anode stream

%weight fractions of other species
w_H2O = 1 - w_H2;
w_N2 = 1 - w_O2;

%--------------- Cathode Stream --------------------------

%mole flow of cathode species - mol/s
n_H2O =  m_C*w_H2O*1000/MM_H2O;
n_H2 = m_C*w_H2*1000/MM_H2;

%mole fraction
x_H2O = n_H2O/(n_H2O + n_H2);
x_H2 = 1 - x_H2O;

%concentrations
c_H2O = c_Tc * x_H2O;
c_H2 = c_Tc * x_H2;

%volumetric flow per cell - m^3/s
V_H2O = (m_C*w_H2O*1000/MM_H2O)*R*T_C/Ppa/num_cells; 
V_H2 = (m_C*w_H2*1000/MM_H2)*R*T_C/Ppa/num_cells;

%velocity, m/s
u_C = (V_H2O + V_H2)/(h_C*W_cell);

%--------------- Anode Stream --------------------------

%mole flow of anode species - mol/s
n_O2 =  m_A*w_O2*1000/MM_O2;
n_N2 = m_A*w_N2*1000/MM_N2;

%mole fraction
x_O2 = n_O2/(n_O2 + n_N2);
x_N2 = 1 - x_O2;

%concentrations
c_O2 = c_Ta * x_O2;
c_N2 = c_Ta * x_N2;

%volumetric flow per cell - m^3/s
V_O2 = (m_A*w_O2*1000/MM_O2)*R*T_A/Ppa/num_cells; 
V_N2 = (m_A*w_N2*1000/MM_N2)*R*T_A/Ppa/num_cells;

%velocity, m/s
u_A = (V_O2 + V_N2)/(h_A*W_cell);

== matlab function HTSE_electrolyzer_1MW_DC/1 MWe-DC Electrolyzer Module/ SOEC Cell ==
  data: u_C input; u_A input; c_H2Oin input; c_H2in input; c_O2in input; c_N2in input; T_Cin input; T_Ain input; U input; j input; c_H2O input; c_H2 input; dcdt_H2O output; c_O2 input; c_N2 input; T_C input; dcdt_H2 output; dcdt_O2 output; dcdt_N2 output; T_A input; T_S input; T_I input; dTdt_C output; dTdt_A output; dTdt_S output; dTdt_I output; k_A parameter; k_C parameter; rho_S parameter; rho_I parameter; lam_I parameter; lam_S parameter; Cp_I parameter; Cp_S parameter; eps_I parameter; eps_S parameter; dx_cell parameter; h_I parameter; h_S parameter; h_A parameter; h_C parameter; sig parameter; F parameter; n_cell parameter; u_C output; u_A output; MM_H2O parameter; MM_H2 parameter; MM_N2 parameter; MM_O2 parameter
function [dcdt_H2O,dcdt_H2,dcdt_O2,dcdt_N2,dTdt_C,dTdt_A,dTdt_S,dTdt_I, u_C, u_A]...
    = HTSEelectrolyzer(u_C, u_A,...
    c_H2Oin,c_H2in,c_O2in,c_N2in,T_Cin, T_Ain, U, j,c_H2O, c_H2,c_O2,c_N2,T_C,T_A,T_S,T_I,...
    k_A, k_C, rho_S, rho_I,lam_I, lam_S, Cp_I, Cp_S, eps_I, eps_S, dx_cell, h_I, h_S, h_A, h_C, sig, F, n_cell,...
    MM_H2O, MM_H2, MM_N2, MM_O2)

%% Cathode Stream Properties
% Get properties that depend on temperature and concentration
%get properties of H2O and H2
[rho_H2O, mu_H2O, k_H2O, C_H2O] = water((T_Cin+T_C(end))/2);
[rho_H2, mu_H2, k_H2, C_H2] = hydrogen((T_Cin+T_C(end))/2);

%avg mole fractions
x_H2O = ((c_H2Oin + c_H2O(end))/2)/( (c_H2Oin + c_H2O(end))/2 + (c_H2in + c_H2(end))/2 );
x_H2 = 1 - x_H2O;

%avg weight fractions
w_H2O = x_H2O * (MM_H2O/(x_H2O*MM_H2O + x_H2*MM_H2) );
w_H2 = 1 - w_H2O;

%use weight fractions for mixing of properties
[rho_C, ~, lam_C, Cp_C] = prop_mix(rho_H2O, rho_H2, mu_H2O, mu_H2, k_H2O, k_H2, C_H2O, C_H2, w_H2O, w_H2);

%% Anode Stream Properties
% Get properties that depend on temperature and concentration

%get properties of O2 and N2
[rho_O2, mu_O2, k_O2, C_O2] = oxygen((T_Ain+T_A(end))/2);
[rho_N2, mu_N2, k_N2, C_N2] = nitrogen((T_Ain+T_A(end))/2);

%avg mole fractions
x_O2 = ((c_O2in + c_O2(end))/2)/( (c_O2in + c_O2(end))/2 + (c_N2in + c_N2(end))/2 );
x_N2 = 1 - x_O2;

%avg weight fractions
w_O2 = x_O2 * (MM_O2/(x_O2*MM_O2 + x_N2*MM_N2) );
w_N2 = 1 - w_O2;

%use weight fractions for mixing of properties
[rho_A, ~, lam_A, Cp_A] = prop_mix(rho_O2, rho_N2, mu_O2, mu_N2, k_O2, k_N2, C_O2, C_N2, w_O2, w_N2);

%% Enthalpy and Rate of Rxn
%initialize enthalpy and rate of reaction
H = zeros(size(c_H2O));
Rrxn = zeros(size(j));

%Find local rate of reaction and heat of reaction
for i = 1:n_cell
    %Interpolation from CoolProp Data
    H(i) = 6214.1*log(T_S(i)) + 204987; %J/mol H2O, enthalpy of reaction at 5 bar
    Rrxn(i) = j(i)/(2*F); %mol/(s*m^2), local reaction rate
end

%% Mass Balances

%For mass and energy balance see detail: Qiong Cai et. al.: Modelling the dynamic
%resonse of a solid oxide steam electrolyzer

%=========================================================================%
%Mass Balance
%Accounts for advective transport and reaction
%Upwind spatial finite difference mixed with central difference using 
%Flux limiters to minimize numerical diffusion

%initializing each mass bal derivatives as zero to define size of each column vector
dcdt_H2O = zeros(size(c_H2O));
dcdt_H2 = zeros(size(c_H2));
dcdt_O2 = zeros(size(c_O2));
dcdt_N2 = zeros(size(c_N2));

F_c_H2O = zeros(size(c_H2O));
F_c_H2 = zeros(size(c_H2));
F_c_O2 = zeros(size(c_O2));
F_c_N2 = zeros(size(c_N2));


%Flux Limiters: calculalate the flux for each concentration
%Can change the limiter method from upwind, but had best stability with upwind
method = "UPWIND";
F_c_H2O = -Flux_Limiter(c_H2O, c_H2Oin, u_C, dx_cell, method);
F_c_H2 = -Flux_Limiter(c_H2, c_H2in, u_C, dx_cell, method);
F_c_O2 = -Flux_Limiter(c_O2, c_O2in, u_A, dx_cell, method);
F_c_N2 = -Flux_Limiter(c_N2, c_N2in, u_A, dx_cell, method);


%Mass balance equations - Flux limiters use B.C's that concentations before
%and after end of cell are what enters/exits respectively

for i = 1:n_cell
%     
%     Direct upwind implementation
%     if i == 1
%         F_c_H2O(i) = u_C*(c_H2Oin - c_H2O(i))/dx_cell;
%         F_c_H2(i)  = u_C*(c_H2in  - c_H2(i))/dx_cell;
%         F_c_O2(i)  = u_A*(c_O2in  - c_O2(i))/dx_cell;
%         F_c_N2(i)  = u_A*(c_N2in  - c_N2(i))/dx_cell;
%     else
%         F_c_H2O(i) = u_C*(c_H2O(i-1) - c_H2O(i))/dx_cell;
%         F_c_H2(i)  = u_C*(c_H2(i-1)  - c_H2(i))/dx_cell;
%         F_c_O2(i)  = u_A*(c_O2(i-1)  - c_O2(i))/dx_cell;
%         F_c_N2(i)  = u_A*(c_N2(i-1)  - c_N2(i))/dx_cell;
%     end
    %Water
    dcdt_H2O(i) = F_c_H2O(i) - Rrxn(i)/h_C;
    %Hydrogen
    dcdt_H2(i) = F_c_H2(i) + Rrxn(i)/h_C;
    %Oxygen
    dcdt_O2(i) = F_c_O2(i) + Rrxn(i)/(2*h_A);
    %Nitrogen
    dcdt_N2(i) = F_c_N2(i);
end

%% Energy Balance
%=========================================================================%


%initializing energy bal deriviatives as zero to define size of each column vector
%cathode stream
dTdt_C = zeros(size(T_C));
%anode stream
dTdt_A = zeros(size(T_A));
%solid structure (contains cathode, anode and electrolyte)
dTdt_S = zeros(size(T_S));
%interconnect
dTdt_I = zeros(size(T_I));


F_T_C = zeros(size(T_C));
F_T_A = zeros(size(T_A));

%Flux Limiters: fluxes for cathode and anode temperatures
% method = "KOREN";
F_T_C = -Flux_Limiter(T_C, T_Cin, u_C, dx_cell, method);
F_T_A = -Flux_Limiter(T_A, T_Ain, u_A, dx_cell, method);

for i = 1:n_cell
    
%     if i == 1
%         F_T_C(i) = u_C*(T_Cin - T_C(i))/dx_cell;
%         F_T_A(i) = u_A*(T_Ain - T_A(i))/dx_cell;
%     else
%         F_T_C(i) = u_C*(T_C(i-1) - T_C(i))/dx_cell;
%         F_T_A(i) = u_A*(T_A(i-1) - T_A(i))/dx_cell;
%     end

    %cathode stream
    dTdt_C(i) = F_T_C(i) + k_C/(rho_C*Cp_C*h_C)*(T_S(i) + T_I(i) - 2*T_C(i));
    %anode stream
    dTdt_A(i) = F_T_A(i) + k_A/(rho_A*Cp_A*h_A)*(T_S(i) + T_I(i) - 2*T_A(i));
end


%first node for solid structure and interface uses neumann BC = 0 at front and
%end of the cell. All use central difference scheme

%T_Sin = (T_Cin + T_Ain)/2;
%T_Iin = T_Sin;

%solid structure (contains cathode, anode and electrolyte) 1st node: w/ neumann BC sub
dTdt_S(1) =  lam_S/(rho_S*Cp_S)*(T_S(2) - T_S(1))/dx_cell^2 -... 
k_C/(rho_S*Cp_S*h_S)*(T_S(1) - T_C(1)) - k_A/(rho_S*Cp_S*h_S)*(T_S(1) - T_A(1)) -...
2/(rho_S*Cp_S*h_S)*(sig*(T_S(1)^4 - T_I(1)^4))/(1/eps_S + 1/eps_I -1) +...
1/(rho_S*Cp_S*h_S)*(-H(1)*Rrxn(1) + j(1)*U);

%interconnect 1st node: w/ neumann BC sub
dTdt_I(1) = lam_I/(rho_I*Cp_I)*(T_I(2) - T_I(1))/dx_cell^2 -... 
k_C/(rho_I*Cp_I*h_I)*(T_I(1) - T_C(1)) - k_A/(rho_I*Cp_I*h_I)*(T_I(1) - T_A(1)) +...
2/(rho_I*Cp_I*h_I)*(sig*(T_S(1)^4 - T_I(1)^4))/(1/eps_S + 1/eps_I -1);


%central differnce for all internal nodes - no special conditions
for i = 2:n_cell-1
    %solid structure (contains cathode, anode and electrolyte)
    dTdt_S(i) = lam_S/(rho_S*Cp_S)*(T_S(i+1) - 2*T_S(i)+ T_S(i-1))/dx_cell^2 -... 
    k_C/(rho_S*Cp_S*h_S)*(T_S(i) - T_C(i)) - k_A/(rho_S*Cp_S*h_S)*(T_S(i) - T_A(i)) -...
    2/(rho_S*Cp_S*h_S)*(sig*(T_S(i)^4 - T_I(i)^4))/(1/eps_S + 1/eps_I -1) +...
    1/(rho_S*Cp_S*h_S)*(-H(i)*Rrxn(i) + j(i)*U);
    %interconnect
    dTdt_I(i) = lam_I/(rho_I*Cp_I)*(T_I(i+1) - 2*T_I(i)+ T_I(i-1))/dx_cell^2 -... 
    k_C/(rho_I*Cp_I*h_I)*(T_I(i) - T_C(i)) - k_A/(rho_I*Cp_I*h_I)*(T_I(i) - T_A(i)) +...
    2/(rho_I*Cp_I*h_I)*(sig*(T_S(i)^4 - T_I(i)^4))/(1/eps_S + 1/eps_I -1);
end

%Solid structure last node using Neumann B.Cs
dTdt_S(n_cell) =  lam_S/(rho_S*Cp_S)*(T_S(n_cell-1) - T_S(n_cell))/dx_cell^2 -... 
k_C/(rho_S*Cp_S*h_S)*(T_S(n_cell) - T_C(n_cell)) - k_A/(rho_S*Cp_S*h_S)*(T_S(n_cell) - T_A(n_cell)) -...
2/(rho_S*Cp_S*h_S)*(sig*(T_S(n_cell)^4 - T_I(n_cell)^4))/(1/eps_S + 1/eps_I -1) +...
1/(rho_S*Cp_S*h_S)*(-H(n_cell)*Rrxn(n_cell) + j(n_cell)*U);

%Interconnect last node using Neumann B.Cs
dTdt_I(n_cell) = lam_I/(rho_I*Cp_I)*(T_I(n_cell-1) - T_I(n_cell))/dx_cell^2 -... 
k_C/(rho_I*Cp_I*h_I)*(T_I(n_cell) - T_C(n_cell)) - k_A/(rho_I*Cp_I*h_I)*(T_I(n_cell) - T_A(n_cell)) +...
2/(rho_I*Cp_I*h_I)*(sig*(T_S(n_cell)^4 - T_I(n_cell)^4))/(1/eps_S + 1/eps_I -1);

end
